simulink model "simulation_1"  (R2023b)
settings: Solver=VariableStepAuto  StartTime=0.0  StopTime=10.0  RelTol=1e-3
undefined symbols (not defined in the file): j
settings Model: Creator=nurbi  LastModifiedBy=nurbi

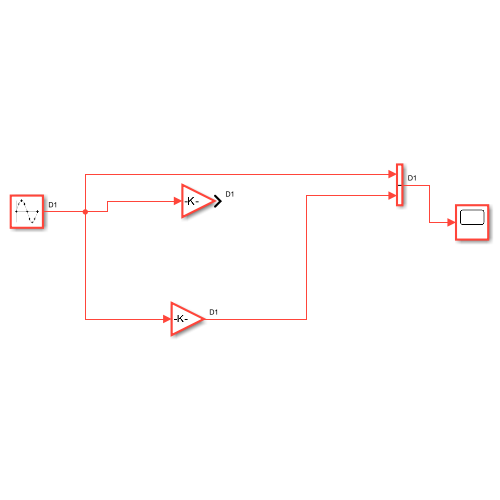
[thumbnail: Simulink's stored preview of the top-level diagram]
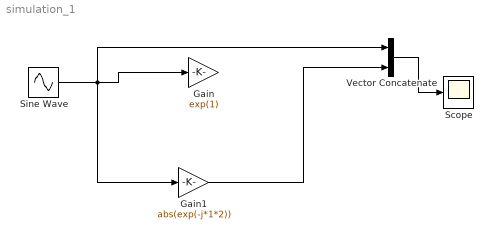
== system simulation_1 ==
  Gain : Gain  Gain=exp(1)
  Gain1 : Gain  Gain=abs(exp(-j*1*2))
  Scope : Scope
  Sine Wave : Sin  SineType=Sample based  Frequency=10  Samples=1000  SampleTime=0.001
  Vector Concatenate : Concatenate
  wires:
  Vector Concatenate/1 -> Scope/1
  Sine Wave/1 -> Vector Concatenate/1, Gain1/1, Gain/1
  Gain1/1 -> Vector Concatenate/2
